simulink model "ship_template2"  (R2020b)
settings: Solver=ode4  StartTime=0  StopTime=30  FixedStep=1e-2  RelTol=1e-3  AbsTol=1e-6
model workspace: external: MATLAB File points.m (data not in the file)
undefined symbols (not defined in the file or in its folder): magnitude
libraries: pid_lib x2, simulink x2
settings Model: ExtModeTrigMode=oneshot  ExtModeArmWhenConnect=off  Creator=jerome  LastModifiedBy=alexs
settings SolverCC: AutoScaleAbsTol=off
settings DataIOCC: SaveFormat=Array  SignalLoggingSaveFormat=ModelDataLogs  ReturnWorkspaceOutputs=off
settings OptimizationCC: BlockReduction=off  BooleanDataType=off  ExpressionDepthLimit=2147483647  InitFltsAndDblsToZero=on  LifeSpan=inf
settings DebuggingCC: SaveWithParameterizedLinksMsg=none  UnderspecifiedInitializationDetection=Classic  MergeDetectMultiDrivingBlocksExec=none  SignalResolutionControl=TryResolveAllWithWarning  MultiTaskDSMMsg=warning  MultiTaskCondExecSysMsg=none  FcnCallInpInsideContextMsg=warning  StateNameClashWarn=warning  SFUnexpectedBacktrackingDiag=warning  SFNoUnconditionalDefaultTransitionDiag=warning  SFExecutionAtInitializationDiag=none  ArithmeticOperatorsInVariantConditions=warning
settings HardwareCC: ProdBitPerPointer=32  ProdBitPerSizeT=32  ProdBitPerPtrDiffT=32  ProdLargestAtomicFloat=None  ProdIntDivRoundTo=Undefined  ProdEndianess=Unspecified  ProdWordSize=32  ProdHWDeviceType=32-bit Generic  TargetUnknown=on
settings ModelReferenceCC: PropagateSignalLabelsOutOfModel=off
settings SFSimCC: SimUseLocalCustomCode=off  CustomCodeUndefinedFunction=UseInterfaceOnly
settings RTWCC: RTWUseLocalCustomCode=off
settings CodeAppCC: StateflowObjectComments=on
settings GRTTargetCC: TargetFcnLib=ansi_tfl_tmw.mat  TargetLangStandard=C89/C90 (ANSI)  ModelReferenceCompliant=off  CombineOutputUpdateFcns=off  MatFileLogging=off  GRTInterface=on
settings ConfigComp: CovMetricSettings=dw  CovSaveCumulativeToWorkspaceVar=on  CovSaveSingleToWorkspaceVar=on  CovExternalEMLEnable=off

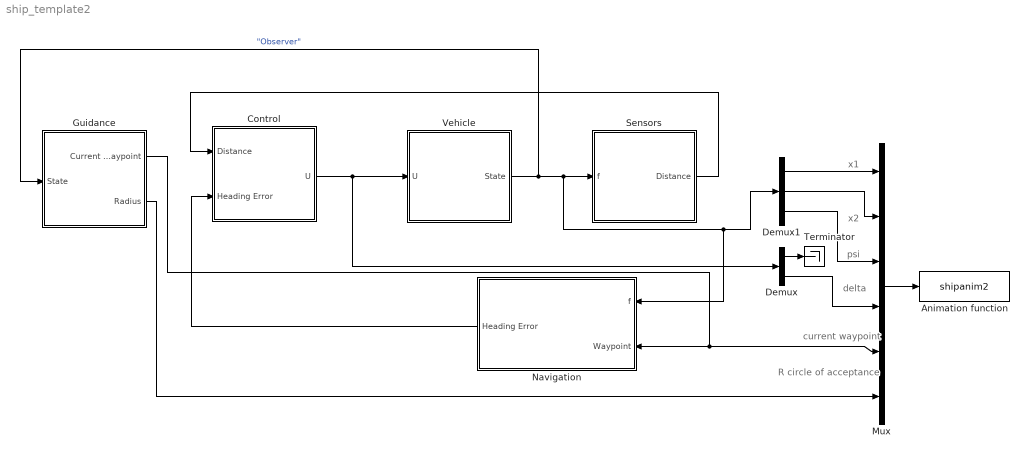
== system ship_template2 ==
  note: R circle of acceptance
  note: delta
  note: psi
  note: x2
  note: x1
  note: current waypoint
  Animation function : S-Function  FunctionName=shipanim2  SFunctionDeploymentMode=off  EnableBusSupport=off
  Control : Subsystem
  Demux : Demux  Outputs=2
  Demux1 : Demux  Outputs=3
  Guidance : Subsystem
  Mux : Mux  Inputs=6
  Navigation : Subsystem
  Sensors : Subsystem
  Terminator : Terminator
  Vehicle : Subsystem
  wires:
  Mux/1 -> Animation function/1
  Sensors/1(Distance) -> Control/1(Distance)
  Control/1(U) -> Vehicle/1(U), Demux/1
  Navigation/1(Heading Error) -> Control/2(Heading Error)
  Vehicle/1(State) -> Guidance/1(State), Sensors/1(f), Navigation/1(f), Demux1/1  "\"Observer\""
  Demux/2 -> Mux/4
  Demux/1 -> Terminator/1
  Demux1/1 -> Mux/1
  Demux1/2 -> Mux/2
  Demux1/3 -> Mux/3
  Guidance/2(Radius) -> Mux/6
  Guidance/1(Current Waypoint) -> Mux/5, Navigation/2(Waypoint)

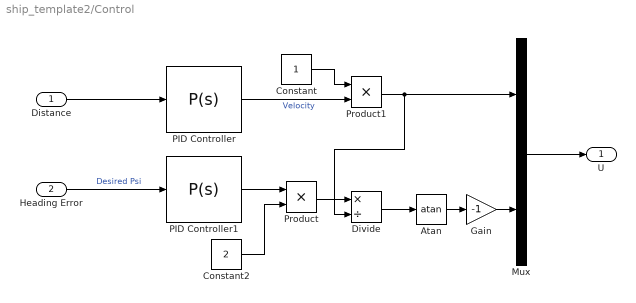
== system ship_template2/Control ==
  Distance : Inport
  Heading Error : Inport  Port=2
  Atan : Trigonometry  Operator=atan
  Constant : Constant
  Constant2 : Constant  Value=2
  Divide : Product  Inputs=*/
  Gain : Gain  Gain=-1
  Mux : Mux  Inputs=2
  PID Controller : pid_lib/PID Controller  Controller=P  Form=Parallel  TimeDomain=Continuous-time  UseExternalTs=off  SampleTime=-1  IntegratorMethod=Forward Euler  FilterMethod=Forward Euler  ControllerParametersSource=internal  P=0.25  I=0.05  D=.5  UseFilter=on  N=100  TunerSelectOption=Transfer Function Based (PID Tuner App)  InitialConditionSource=internal  InitialConditionForIntegrator=0  InitialConditionForFilter=0  DifferentiatorICPrevScaledInput=0  ExternalReset=none  TrackingMode=off  Kt=1  LimitOutput=off  SatLimitsSource=internal  UpperSaturationLimit=inf  LowerSaturationLimit=-inf  LinearizeAsGain=on  AntiWindupMode=none  Kb=1  POutMin=[]  POutMax=[]  IOutMin=[]  IOutMax=[]  DOutMin=[]  DOutMax=[]  NOutMin=[]  NOutMax=[]  SumOutMin=[]  SumOutMax=[]  SaturationOutMin=[]  SaturationOutMax=[]  PParamMin=[]  PParamMax=[]  IParamMin=[]  IParamMax=[]  DParamMin=[]  DParamMax=[]  NParamMin=[]  NParamMax=[]  KbParamMin=[]  KbParamMax=[]  KtParamMin=[]  KtParamMax=[]  KbOutMin=[]  KbOutMax=[]  KtOutMin=[]  KtOutMax=[]  IntegratorOutMin=[]  IntegratorOutMax=[]  FilterOutMin=[]  FilterOutMax=[]  SumI1OutMin=[]  SumI1OutMax=[]  SumI2OutMin=[]  SumI2OutMax=[]  SumI3OutMin=[]  SumI3OutMax=[]  SumI4OutMin=[]  SumI4OutMax=[]  SumDOutMin=[]  SumDOutMax=[]  DifferentiatorOutMin=[]  DifferentiatorOutMax=[]  FilterDiffOutCoefMin=[]  FilterDiffOutCoefMax=[]  ReciprocalOutMin=[]  ReciprocalOutMax=[]  SumDenOutMin=[]  SumDenOutMax=[]  SumNumOutMin=[]  SumNumOutMax=[]  DivideOutMin=[]  DivideOutMax=[]  UdiffTsProdOutMin=[]  UdiffTsProdOutMax=[]  NTsProdOutMin=[]  NTsProdOutMax=[]  UintegralTsProdOutMin=[]  UintegralTsProdOutMax=[]  UngainTsProdOutMin=[]  UngainTsProdOutMax=[]  IntegratorContinuousStateAttributes=''  IntegratorStateMustResolveToSignalObject=off  IntegratorRTWStateStorageClass=Auto  FilterContinuousStateAttributes=''  FilterStateMustResolveToSignalObject=off  FilterRTWStateStorageClass=Auto  ParallelPVariant=InternalParameters  IdealPVariant=Disabled  IVariant=Disabled  DVariant=Disabled  IntegratorVariant=Disabled  SatVariant=Disabled  AWVariant=Disabled  PCopyVariant=Disabled  TRVariant=Disabled  FdbkBlocksVariant=Forward  IdealPFdbkVariant=Disabled  SatFdbkVariant=Disabled  DerivativeFilterVariant=Disabled  NVariant=Disabled  NCopyVariant=Disabled_SignalSpec  FilterICVariant=Disabled  IntegratorICVariant=Disabled  ExternalResetVariant=Disabled  TRSumVariant=Passthrough  SumFdbkVariant=Disabled  SumVariant=Passthrough_P  TsampFilterVariant=InternalTs  TsampNgainVariant=Passthrough  TsampIntegralVariant=Disabled_SignalSpec  ExternalSaturationOutDataTypeStr=Inherit: Same as second input
  PID Controller1 : pid_lib/PID Controller  Controller=P  Form=Parallel  TimeDomain=Continuous-time  UseExternalTs=off  SampleTime=-1  IntegratorMethod=Forward Euler  FilterMethod=Forward Euler  ControllerParametersSource=internal  P=5  I=1  D=0  UseFilter=on  N=100  TunerSelectOption=Transfer Function Based (PID Tuner App)  InitialConditionSource=internal  InitialConditionForIntegrator=0  InitialConditionForFilter=0  DifferentiatorICPrevScaledInput=0  ExternalReset=none  TrackingMode=off  Kt=1  LimitOutput=off  SatLimitsSource=internal  UpperSaturationLimit=inf  LowerSaturationLimit=-inf  LinearizeAsGain=on  AntiWindupMode=none  Kb=1  POutMin=[]  POutMax=[]  IOutMin=[]  IOutMax=[]  DOutMin=[]  DOutMax=[]  NOutMin=[]  NOutMax=[]  SumOutMin=[]  SumOutMax=[]  SaturationOutMin=[]  SaturationOutMax=[]  PParamMin=[]  PParamMax=[]  IParamMin=[]  IParamMax=[]  DParamMin=[]  DParamMax=[]  NParamMin=[]  NParamMax=[]  KbParamMin=[]  KbParamMax=[]  KtParamMin=[]  KtParamMax=[]  KbOutMin=[]  KbOutMax=[]  KtOutMin=[]  KtOutMax=[]  IntegratorOutMin=[]  IntegratorOutMax=[]  FilterOutMin=[]  FilterOutMax=[]  SumI1OutMin=[]  SumI1OutMax=[]  SumI2OutMin=[]  SumI2OutMax=[]  SumI3OutMin=[]  SumI3OutMax=[]  SumI4OutMin=[]  SumI4OutMax=[]  SumDOutMin=[]  SumDOutMax=[]  DifferentiatorOutMin=[]  DifferentiatorOutMax=[]  FilterDiffOutCoefMin=[]  FilterDiffOutCoefMax=[]  ReciprocalOutMin=[]  ReciprocalOutMax=[]  SumDenOutMin=[]  SumDenOutMax=[]  SumNumOutMin=[]  SumNumOutMax=[]  DivideOutMin=[]  DivideOutMax=[]  UdiffTsProdOutMin=[]  UdiffTsProdOutMax=[]  NTsProdOutMin=[]  NTsProdOutMax=[]  UintegralTsProdOutMin=[]  UintegralTsProdOutMax=[]  UngainTsProdOutMin=[]  UngainTsProdOutMax=[]  IntegratorContinuousStateAttributes=''  IntegratorStateMustResolveToSignalObject=off  IntegratorRTWStateStorageClass=Auto  FilterContinuousStateAttributes=''  FilterStateMustResolveToSignalObject=off  FilterRTWStateStorageClass=Auto  ParallelPVariant=InternalParameters  IdealPVariant=Disabled  IVariant=Disabled  DVariant=Disabled  IntegratorVariant=Disabled  SatVariant=Disabled  AWVariant=Disabled  PCopyVariant=Disabled  TRVariant=Disabled  FdbkBlocksVariant=Forward  IdealPFdbkVariant=Disabled  SatFdbkVariant=Disabled  DerivativeFilterVariant=Disabled  NVariant=Disabled  NCopyVariant=Disabled_SignalSpec  FilterICVariant=Disabled  IntegratorICVariant=Disabled  ExternalResetVariant=Disabled  TRSumVariant=Passthrough  SumFdbkVariant=Disabled  SumVariant=Passthrough_P  TsampFilterVariant=InternalTs  TsampNgainVariant=Passthrough  TsampIntegralVariant=Disabled_SignalSpec  ExternalSaturationOutDataTypeStr=Inherit: Same as second input
  Product : Product
  Product1 : Product
  U : Outport
  wires:
  Mux/1 -> U/1
  PID Controller/1 -> Product1/2  "Velocity"
  Constant/1 -> Product1/1
  Product/1 -> Divide/1
  Distance/1 -> PID Controller/1
  PID Controller1/1 -> Product/1
  Heading Error/1 -> PID Controller1/1  "Desired Psi"
  Divide/1 -> Atan/1
  Constant2/1 -> Product/2
  Atan/1 -> Gain/1
  Gain/1 -> Mux/2
  Product1/1 -> Divide/2, Mux/1

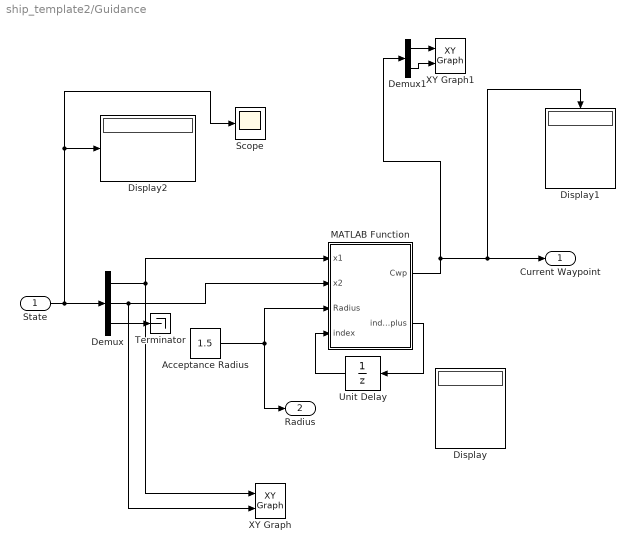
== system ship_template2/Guidance ==
  State : Inport
  Acceptance Radius : Constant  Value=1.5
  Demux : Demux  Outputs=3
  Demux1 : Demux  Outputs=2
  Display : Display
  Display1 : Display
  Display2 : Display
  MATLAB Function : MATLAB Function  TreatAsAtomicUnit=on
  Scope : Scope
  Terminator : Terminator
  Unit Delay : UnitDelay  SampleTime=-1  HasFrameUpgradeWarning=on
  XY Graph : simulink/Sinks/XY Graph  xmin=-10  xmax=10  ymin=-10  ymax=10  st=-1
  XY Graph1 : simulink/Sinks/XY Graph  xmin=-10  xmax=10  ymin=-10  ymax=10  st=-1
  Current Waypoint : Outport
  Radius : Outport  Port=2
  wires:
  MATLAB Function/1(Cwp) -> Demux1/1, Display1/1, Current Waypoint/1
  Unit Delay/1 -> MATLAB Function/4(index)
  State/1 -> Scope/1, Display2/1, Demux/1
  Demux/3 -> Terminator/1
  Demux/2 -> MATLAB Function/2(x2), XY Graph/2
  Demux/1 -> XY Graph/1, MATLAB Function/1(x1)
  Acceptance Radius/1 -> Radius/1, MATLAB Function/3(Radius)
  Demux1/1 -> XY Graph1/1
  Demux1/2 -> XY Graph1/2
  MATLAB Function/2(index_plus) -> Unit Delay/1

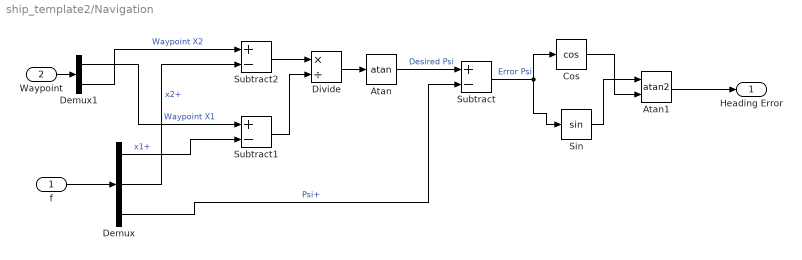
== system ship_template2/Navigation ==
  f : Inport
  Waypoint : Inport  Port=2
  Atan : Trigonometry  Operator=atan
  Atan1 : Trigonometry  Operator=atan2
  Cos : Trigonometry  Operator=cos
  Demux : Demux  Outputs=3
  Demux1 : Demux  Outputs=2
  Divide : Product  Inputs=*/
  Sin : Trigonometry
  Subtract : Sum  Inputs=+-
  Subtract1 : Sum  Inputs=+-
  Subtract2 : Sum  Inputs=+-
  Heading Error : Outport
  wires:
  Divide/1 -> Atan/1
  Demux1/1 -> Subtract1/1  "Waypoint X1"
  Atan/1 -> Subtract/1  "Desired Psi"
  Demux/1 -> Subtract1/2  "x1+"
  Cos/1 -> Atan1/2
  Subtract/1 -> Sin/1, Cos/1  "Error Psi"
  Sin/1 -> Atan1/1
  Atan1/1 -> Heading Error/1
  Subtract1/1 -> Divide/2
  f/1 -> Demux/1
  Demux/2 -> Subtract2/2  "x2+"
  Demux/3 -> Subtract/2  "Psi+"
  Demux1/2 -> Subtract2/1  "Waypoint X2"
  Subtract2/1 -> Divide/1
  Waypoint/1 -> Demux1/1

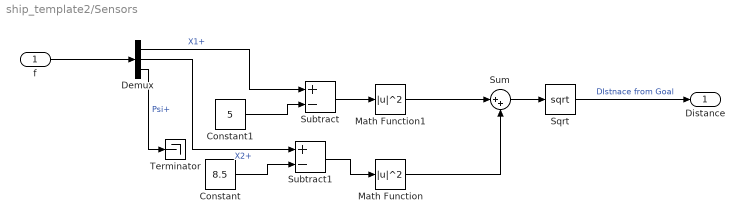
== system ship_template2/Sensors ==
  f : Inport
  Constant : Constant  Value=8.5
  Constant1 : Constant  Value=5
  Demux : Demux  Outputs=3
  Math Function : Math  Operator=magnitude^2  SaturateOnIntegerOverflow=on
  Math Function1 : Math  Operator=magnitude^2  SaturateOnIntegerOverflow=on
  Sqrt : Sqrt  SaturateOnIntegerOverflow=on
  Subtract : Sum  Inputs=+-
  Subtract1 : Sum  Inputs=+-
  Sum : Sum  Inputs=|++
  Terminator : Terminator
  Distance : Outport
  wires:
  Sum/1 -> Sqrt/1
  Constant1/1 -> Subtract/2
  Subtract1/1 -> Math Function/1
  Math Function/1 -> Sum/2
  Subtract/1 -> Math Function1/1
  Demux/1 -> Subtract/1  "X1+"
  Constant/1 -> Subtract1/2
  f/1 -> Demux/1
  Math Function1/1 -> Sum/1
  Demux/2 -> Subtract1/1  "X2+"
  Sqrt/1 -> Distance/1  "DIstnace from Goal"
  Demux/3 -> Terminator/1  "Psi+"

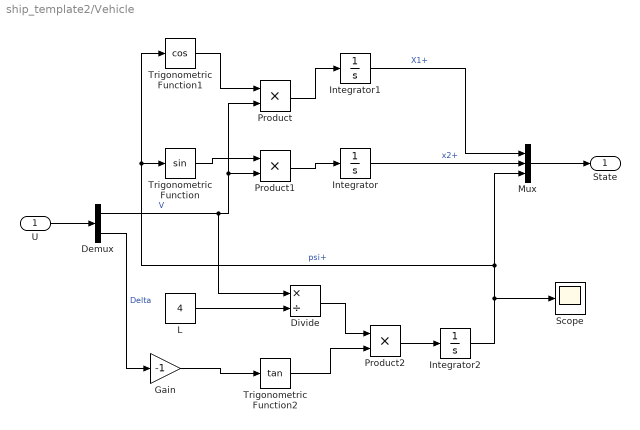
== system ship_template2/Vehicle ==
  U : Inport
  Demux : Demux  Outputs=2
  Divide : Product  Inputs=*/
  Gain : Gain  Gain=-1
  Integrator : Integrator  InitialCondition=-8
  Integrator1 : Integrator  InitialCondition=-11
  Integrator2 : Integrator  InitialCondition=0
  L : Constant  Value=4
  Mux : Mux  Inputs=3
  Product : Product
  Product1 : Product
  Product2 : Product
  Scope : Scope
  Trigonometric Function : Trigonometry
  Trigonometric Function1 : Trigonometry  Operator=cos
  Trigonometric Function2 : Trigonometry  Operator=tan
  State : Outport
  wires:
  Trigonometric Function1/1 -> Product/1
  Trigonometric Function/1 -> Product1/1
  Divide/1 -> Product2/1
  L/1 -> Divide/2
  Demux/2 -> Gain/1  "Delta"
  Integrator1/1 -> Mux/1  "X1+"
  U/1 -> Demux/1
  Product1/1 -> Integrator/1
  Integrator/1 -> Mux/2  "x2+"
  Demux/1 -> Divide/1, Product/2, Product1/2  "V"
  Product/1 -> Integrator1/1
  Gain/1 -> Trigonometric Function2/1
  Trigonometric Function2/1 -> Product2/2
  Product2/1 -> Integrator2/1
  Mux/1 -> State/1
  Integrator2/1 -> Mux/3, Trigonometric Function1/1, Trigonometric Function/1, Scope/1  "psi+"

== matlab function ship_template2/Guidance/MATLAB Function ==
  data: x1 input; x2 input; Radius input; Cwp output double; index input; index_plus output
function [Cwp, index_plus]  = fcn(x1, x2, Radius, index)

%% Using spline function
% x = [-10 0 5]
% y = [-8 8 8]
% xx = -10:.5:5;
% yy = spline(x,y,xx)
% plot(x,y,'o',xx,yy)

%% Using ploynomial function

% Start and end point
waypoint_index = 0

waypoints_x = [-10 5 -5]
waypoints_y = [-8 8.5 5]



x = [-10 5];
y = [-8 8.5];

vd0 = 50;
vyd1 = 0;

vd1 = 30;
vyd0 = 0;

[Cwp, index_plus] = poly_waypoints(x1, x2, Radius, index, x, y, vd0, vyd1, vd1, vyd0)

if 

function [Cwp, index_plus] = poly_waypoints(x1, x2, Radius, index, x, y, vd0, vyd1, vd1, vyd0)

    xv_vec = [x(1);
              vd0;
              x(2);
              vd1];
    yv_vec = [y(1);
              vyd0;
              y(2);
              vyd1];

    alpha_x = alpha(xv_vec)
    alpha_y = alpha(yv_vec)

    % sig = sqrt((x1 - x(1))^2 + (x2-y(1))^2) / sqrt((x(2) - x(1))^2 + (y(2)-y(1))^2)
    sig = index
    x_value = poly(alpha_x, sig);
    y_value = poly(alpha_y, sig);

    %% Checks whether ship is within range of waypoint. If yes, it switches to next.
    index_plus = index;
    if (in_range(x1,x_value, x2, y_value, Radius) == 1)
        if (sqrt( (x1-x(2))^2 + (x2-y(2))^2)) >= Radius
            index_plus = index + 0.01;
        end    
    end

    %%
    data = [x_value; y_value]
    Cwp = data;
end

%% Support functions
function bool = in_range(x_a, x_b, y_a, y_b, Radius)
    bool = 0;
    range = sqrt( (x_a-x_b)^2 + (y_a-y_b)^2);
    if range <= Radius
        bool = 1;             
    end
end

function poly = poly(alpha, sigma)
    poly = alpha(1)+alpha(2)*sigma+alpha(3)*sigma^2+alpha(4)*sigma^3;
end
function alpha = alpha(xv_vec)
    b_vec = [b(0)'; 
            b_deriv(0)';
            b(1)';
            b_deriv(1)'];

    alpha = inv(b_vec)*xv_vec;
end
function b = b(sigma)
    b = [1 sigma sigma^2 sigma^3]';
end
function b_deriv = b_deriv(sigma)
    b_deriv = [0 1 2*sigma 3*sigma^2]';
end
end
